simulink library "libMdl_crossProdMat"  (R2019b)
settings: Solver=VariableStepAuto  StartTime=0.0  StopTime=10.0  RelTol=1e-3
settings Model: Creator=hwinter  LastModifiedBy=Hanno
settings DataIOCC: ReturnWorkspaceOutputs=off
settings DebuggingCC: ArithmeticOperatorsInVariantConditions=warning
settings SFSimCC: SimUseLocalCustomCode=off  CustomCodeUndefinedFunction=UseInterfaceOnly
settings RTWCC: RTWUseLocalCustomCode=off

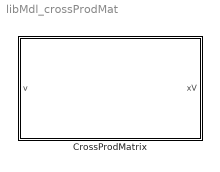
== system libMdl_crossProdMat ==
  CrossProdMatrix : Subsystem
      mask Display:
      | color('black')
      | port_label('input', 1, 'v', 'texmode','on')
      | port_label('output', 1, '[v\times]', 'texmode','on')

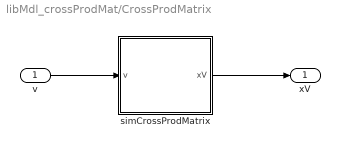
== system libMdl_crossProdMat/CrossProdMatrix ==
  v : Inport
  simCrossProdMatrix : MATLAB Function  TreatAsAtomicUnit=on
  xV : Outport  VectorParamsAs1DForOutWhenUnconnected=off
  wires:
  v/1 -> simCrossProdMatrix/1(v)
  simCrossProdMatrix/1(xV) -> xV/1

== matlab function libMdl_crossProdMat/CrossProdMatrix/simCrossProdMatrix ==
  data: v input; xV output
function xV = simCrossProdMatrix(v)

if length(v) ~= 3
    error('simCrossProdMatrix: Input vector has wrong dimension!');
end % if

xV = [ ...
           0, -v(3),  v(2); ... 
        v(3),     0, -v(1); ...
       -v(2),  v(1),     0  ...
     ];

end % function
